simulink library "WECSim_Lib"  (R2014b)
settings: Solver=ode45  StartTime=0.0  StopTime=10.0  RelTol=1e-3
undefined symbols (not defined in the file): body, constraint, pto, simu, waves, X, Y, Z
libraries: nesl_utility x107, sm_lib x53
(part 2 of 4)

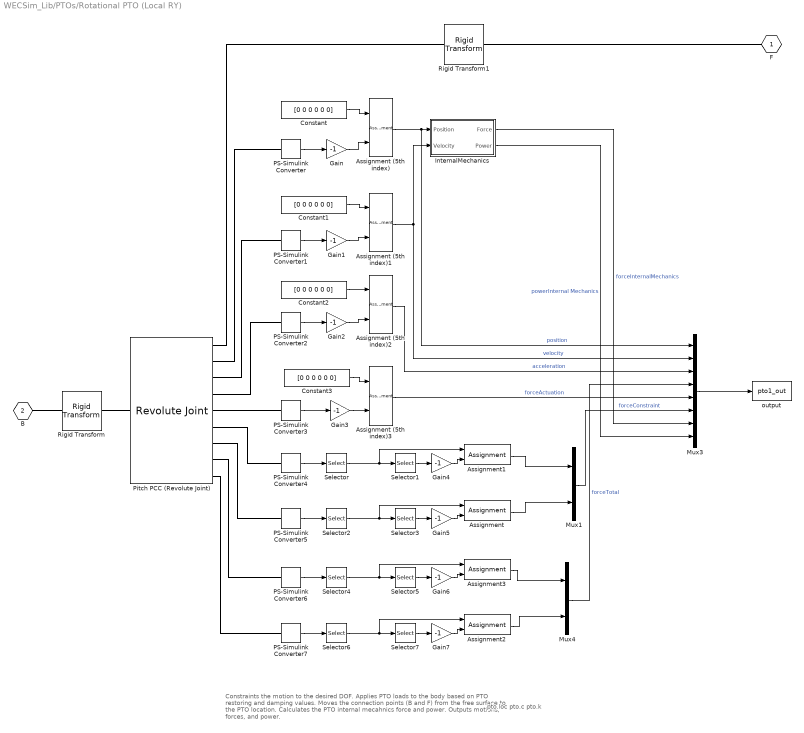
== system WECSim_Lib/PTOs/Rotational PTO (Local RY) ==
  note: Constraints the motion to the desired DOF.
      | Applies PTO loads to the body based on PTO restoring and damping values.
      | Moves the connection points (B and F) from the free surface to the PTO location.
      | Calculates the PTO internal mecahnics force and power.
      | Outputs motions, forces, and power.
  note: pto.loc
      | pto.c
      | pto.k
  Assignment{,1..3} (4 alike) : Assignment  DiagnosticForDimensions=Warning  Indices=2
  "Assignment (5th index) " : Assignment  Indices=5
  Assignment (5th index)1 : Assignment  Indices=5
  Assignment (5th index)2 : Assignment  Indices=5
  Assignment (5th index)3 : Assignment  Indices=5
  Constant{,1..3} (4 alike) : Constant  Value=[0 0 0 0 0 0]
  Gain{,1..7} (8 alike) : Gain  Gain=-1
  InternalMechanics : Subsystem
  Mux1 : Mux  Inputs=2
  Mux3 : Mux  Inputs=8
  Mux4 : Mux  Inputs=2
  PS-Simulink Converter{,1..7} (8 alike) : nesl_utility/PS-Simulink Converter  PhysicalDomain=network_engine_domain  SubClassName=ps_output  LeftPortType=input  RightPortType=output  PseudoPeriodic=off  Frequencies=[]  Unit=1  AffineConversion=off
  Pitch PCC (Revolute Joint) : sm_lib/Joints/Revolute Joint  SenseConstraintForce=on  SenseConstraintForceX=off  SenseConstraintForceY=off  SenseConstraintForceZ=off  SenseConstraintTorque=on  SenseConstraintTorqueX=off  SenseConstraintTorqueY=off  SenseConstraintTorqueZ=off  SenseTotalForce=on  SenseTotalForceX=off  SenseTotalForceY=off  SenseTotalForceZ=off  SenseTotalTorque=on  SenseTotalTorqueX=off  SenseTotalTorqueY=off  SenseTotalTorqueZ=off  CompositeWrenchDir=BaseOnFollower  CompositeWrenchFrame=BaseFrame  EquilibriumPosition=0  EquilibriumPositionUnits=deg  SpringStiffness=pto.k  SpringStiffnessUnits=N*m/rad  DampingCoefficient=pto.c  DampingCoefficientUnits=N*m/(rad/s)  TorqueActuationMode=NoTorque  MotionActuationMode=ComputedMotion  SensePosition=on  SenseVelocity=on  SenseAcceleration=on  SenseTorqueForce=on  PositionTargetValue=0  PositionTargetValueUnits=deg  PositionTargetSpecify=off  PositionTargetPriority=High  VelocityTargetValue=0  VelocityTargetValueUnits=deg/s  VelocityTargetSpecify=off  VelocityTargetPriority=High  BlockFunction=simmechanics.library.joints.revolute_joint
  Rigid Transform : sm_lib/Frames and Transforms/Rigid Transform  TranslationMethod=Cartesian  TranslationLengthUnit=m  TranslationStandardAxis=+Z  TranslationStandardOffset=0  TranslationCartesianOffset=pto.loc  TranslationROffset=0  TranslationROffsetUnits=m  TranslationZOffset=0  TranslationZOffsetUnits=m  TranslationThetaOffset=0  TranslationThetaOffsetUnits=deg  RotationMethod=StandardAxis  RotationAngleUnits=deg  RotationStandardAxis=+X  RotationAngle=90  RotationArbitraryAxis=[0 0 1]  FollAlignAxisA=+X  BaseAlignAxisA=+Y  FollAlignAxisB=+Y  BaseAlignAxisB=+Z  RotationMatrix=[1 0 0; 0 1 0; 0 0 1]  BlockFunction=simmechanics.library.frames_transforms.rigid_transform
  Rigid Transform1 : sm_lib/Frames and Transforms/Rigid Transform  TranslationMethod=Cartesian  TranslationLengthUnit=m  TranslationStandardAxis=+Z  TranslationStandardOffset=0  TranslationCartesianOffset=pto.loc  TranslationROffset=0  TranslationROffsetUnits=m  TranslationZOffset=0  TranslationZOffsetUnits=m  TranslationThetaOffset=0  TranslationThetaOffsetUnits=deg  RotationMethod=StandardAxis  RotationAngleUnits=deg  RotationStandardAxis=+X  RotationAngle=90  RotationArbitraryAxis=[0 0 1]  FollAlignAxisA=+X  BaseAlignAxisA=+Y  FollAlignAxisB=+Y  BaseAlignAxisB=+Z  RotationMatrix=[1 0 0; 0 1 0; 0 0 1]  BlockFunction=simmechanics.library.frames_transforms.rigid_transform
  Selector{,2,4,6} (4 alike) : Selector  InputPortWidth=3  Indices=[1 3 2]
  Selector{1,3,5,7} (4 alike) : Selector  InputPortWidth=3  Indices=[2]
  output : ToWorkspace  VariableName=pto1_out  SaveFormat=Structure With Time  SampleTime=-1
  F : PMIOPort  Port=1  Side=Right
  B : PMIOPort  Port=2  Side=Left
  wires:
  InternalMechanics/2(Power) -> Mux3/8  "powerInternal Mechanics"
  InternalMechanics/1(Force) -> Mux3/7  "forceInternalMechanics"
  Assignment (5th index)3/1 -> Mux3/5  "forceActuation"
  Assignment (5th index)2/1 -> Mux3/3  "acceleration"
  PS-Simulink Converter3/1 -> Gain3/1
  Gain3/1 -> Assignment (5th index)3/2
  Constant3/1 -> Assignment (5th index)3/1
  Gain2/1 -> Assignment (5th index)2/2
  Constant2/1 -> Assignment (5th index)2/1
  PS-Simulink Converter2/1 -> Gain2/1
  Assignment (5th index)1/1 -> InternalMechanics/2(Velocity), Mux3/2  "velocity"
  PS-Simulink Converter1/1 -> Gain1/1
  Gain1/1 -> Assignment (5th index)1/2
  Constant1/1 -> Assignment (5th index)1/1
  "Assignment (5th index) "/1 -> InternalMechanics/1(Position), Mux3/1  "position"
  Gain/1 -> "Assignment (5th index) "/2
  PS-Simulink Converter/1 -> Gain/1
  Constant/1 -> "Assignment (5th index) "/1
  Assignment3/1 -> Mux4/1
  Assignment2/1 -> Mux4/2
  PS-Simulink Converter7/1 -> Selector6/1
  PS-Simulink Converter6/1 -> Selector4/1
  Gain6/1 -> Assignment3/2
  Selector5/1 -> Gain6/1
  Selector4/1 -> Assignment3/1, Selector5/1
  Gain7/1 -> Assignment2/2
  Selector7/1 -> Gain7/1
  Selector6/1 -> Assignment2/1, Selector7/1
  Mux4/1 -> Mux3/4  "forceTotal"
  Mux3/1 -> output/1
  PS-Simulink Converter4/1 -> Selector/1
  PS-Simulink Converter5/1 -> Selector2/1
  Mux1/1 -> Mux3/6  "forceConstraint"
  Assignment1/1 -> Mux1/1
  Assignment/1 -> Mux1/2
  Gain4/1 -> Assignment1/2
  Selector1/1 -> Gain4/1
  Selector/1 -> Selector1/1, Assignment1/1
  Gain5/1 -> Assignment/2
  Selector3/1 -> Gain5/1
  Selector2/1 -> Selector3/1, Assignment/1
  connections:
  PS-Simulink Converter3/LConn1 -- Pitch PCC (Revolute Joint)/RConn5
  PS-Simulink Converter2/LConn1 -- Pitch PCC (Revolute Joint)/RConn4
  Pitch PCC (Revolute Joint)/RConn3 -- PS-Simulink Converter1/LConn1
  Pitch PCC (Revolute Joint)/RConn2 -- PS-Simulink Converter/LConn1
  PS-Simulink Converter4/LConn1 -- Pitch PCC (Revolute Joint)/RConn6
  PS-Simulink Converter5/LConn1 -- Pitch PCC (Revolute Joint)/RConn7
  PS-Simulink Converter6/LConn1 -- Pitch PCC (Revolute Joint)/RConn8
  PS-Simulink Converter7/LConn1 -- Pitch PCC (Revolute Joint)/RConn9
  Pitch PCC (Revolute Joint)/RConn1 -- Rigid Transform1/RConn1
  Pitch PCC (Revolute Joint)/LConn1 -- Rigid Transform/RConn1
  B/RConn1 -- Rigid Transform/LConn1
  F/RConn1 -- Rigid Transform1/LConn1

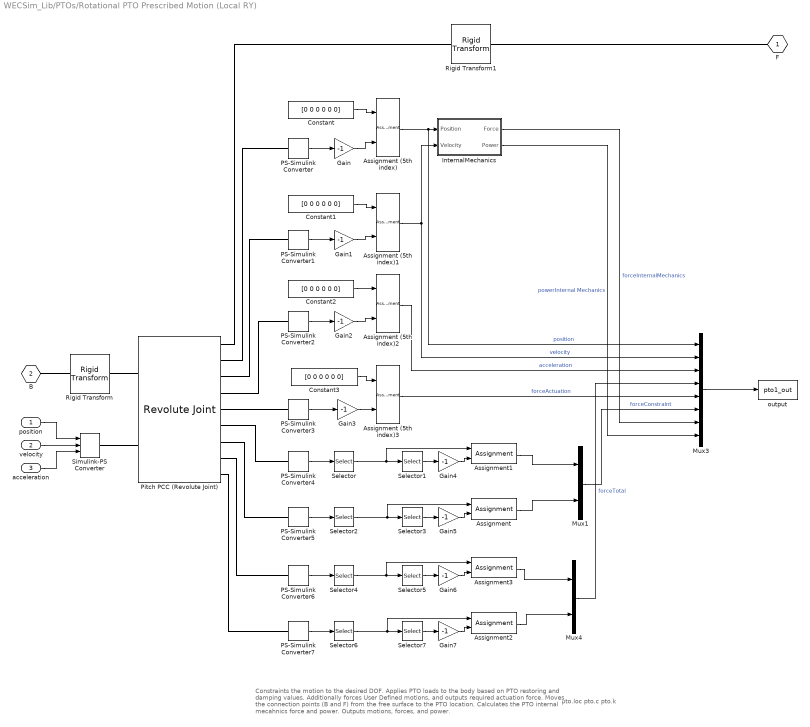
== system WECSim_Lib/PTOs/Rotational PTO Prescribed Motion (Local RY) ==
  note: pto.loc
      | pto.c
      | pto.k
  note: Constraints the motion to the desired DOF.
      | Applies PTO loads to the body based on PTO restoring and damping values.
      | Additionally forces User Defined motions, and outputs required actuation force.
      | Moves the connection points (B and F) from the free surface to the PTO location.
      | Calculates the PTO internal mecahnics force and power.
      | Outputs motions, forces, and power.
  position : Inport
  velocity : Inport  Port=2
  acceleration : Inport  Port=3
  Assignment{,1..3} (4 alike) : Assignment  DiagnosticForDimensions=Warning  Indices=2
  "Assignment (5th index) " : Assignment  Indices=5
  Assignment (5th index)1 : Assignment  Indices=5
  Assignment (5th index)2 : Assignment  Indices=5
  Assignment (5th index)3 : Assignment  Indices=5
  Constant{,1..3} (4 alike) : Constant  Value=[0 0 0 0 0 0]
  Gain{,1..7} (8 alike) : Gain  Gain=-1
  InternalMechanics : Subsystem
  Mux1 : Mux  Inputs=2
  Mux3 : Mux  Inputs=8
  Mux4 : Mux  Inputs=2
  PS-Simulink Converter{,1..7} (8 alike) : nesl_utility/PS-Simulink Converter  PhysicalDomain=network_engine_domain  SubClassName=ps_output  LeftPortType=input  RightPortType=output  PseudoPeriodic=off  Frequencies=[]  Unit=1  AffineConversion=off
  Pitch PCC (Revolute Joint) : sm_lib/Joints/Revolute Joint  SenseConstraintForce=on  SenseConstraintForceX=off  SenseConstraintForceY=off  SenseConstraintForceZ=off  SenseConstraintTorque=on  SenseConstraintTorqueX=off  SenseConstraintTorqueY=off  SenseConstraintTorqueZ=off  SenseTotalForce=on  SenseTotalForceX=off  SenseTotalForceY=off  SenseTotalForceZ=off  SenseTotalTorque=on  SenseTotalTorqueX=off  SenseTotalTorqueY=off  SenseTotalTorqueZ=off  CompositeWrenchDir=BaseOnFollower  CompositeWrenchFrame=BaseFrame  EquilibriumPosition=0  EquilibriumPositionUnits=deg  SpringStiffness=pto.k  SpringStiffnessUnits=N*m/rad  DampingCoefficient=pto.c  DampingCoefficientUnits=N*m/(rad/s)  TorqueActuationMode=ComputedTorque  MotionActuationMode=InputMotion  SensePosition=on  SenseVelocity=on  SenseAcceleration=on  SenseTorqueForce=on  PositionTargetValue=0  PositionTargetValueUnits=deg  PositionTargetSpecify=off  PositionTargetPriority=High  VelocityTargetValue=0  VelocityTargetValueUnits=deg/s  VelocityTargetSpecify=off  VelocityTargetPriority=High  BlockFunction=simmechanics.library.joints.revolute_joint
  Rigid Transform : sm_lib/Frames and Transforms/Rigid Transform  TranslationMethod=Cartesian  TranslationLengthUnit=m  TranslationStandardAxis=+Z  TranslationStandardOffset=0  TranslationCartesianOffset=pto.loc  TranslationROffset=0  TranslationROffsetUnits=m  TranslationZOffset=0  TranslationZOffsetUnits=m  TranslationThetaOffset=0  TranslationThetaOffsetUnits=deg  RotationMethod=StandardAxis  RotationAngleUnits=deg  RotationStandardAxis=+X  RotationAngle=90  RotationArbitraryAxis=[0 0 1]  FollAlignAxisA=+X  BaseAlignAxisA=+Y  FollAlignAxisB=+Y  BaseAlignAxisB=+Z  RotationMatrix=[1 0 0; 0 1 0; 0 0 1]  BlockFunction=simmechanics.library.frames_transforms.rigid_transform
  Rigid Transform1 : sm_lib/Frames and Transforms/Rigid Transform  TranslationMethod=Cartesian  TranslationLengthUnit=m  TranslationStandardAxis=+Z  TranslationStandardOffset=0  TranslationCartesianOffset=pto.loc  TranslationROffset=0  TranslationROffsetUnits=m  TranslationZOffset=0  TranslationZOffsetUnits=m  TranslationThetaOffset=0  TranslationThetaOffsetUnits=deg  RotationMethod=StandardAxis  RotationAngleUnits=deg  RotationStandardAxis=+X  RotationAngle=90  RotationArbitraryAxis=[0 0 1]  FollAlignAxisA=+X  BaseAlignAxisA=+Y  FollAlignAxisB=+Y  BaseAlignAxisB=+Z  RotationMatrix=[1 0 0; 0 1 0; 0 0 1]  BlockFunction=simmechanics.library.frames_transforms.rigid_transform
  Selector{,2,4,6} (4 alike) : Selector  InputPortWidth=3  Indices=[1 3 2]
  Selector{1,3,5,7} (4 alike) : Selector  InputPortWidth=3  Indices=[2]
  Simulink-PS Converter : nesl_utility/Simulink-PS Converter  PhysicalDomain=network_engine_domain  SubClassName=ps_input  LeftPortType=input  RightPortType=output  PseudoPeriodic=off  Frequencies=[]  NoiseDistribution=none  NoiseParameters=[]  Unit=1  AffineConversion=off  InputFiltering=derivs  SimscapeFilterOrder=2  InputFilterTimeConstant=0.001  UdotUserProvided=2
  output : ToWorkspace  VariableName=pto1_out  SaveFormat=Structure With Time  SampleTime=-1
  F : PMIOPort  Port=1  Side=Left
  B : PMIOPort  Port=2  Side=Right
  wires:
  position/1 -> Simulink-PS Converter/1
  velocity/1 -> Simulink-PS Converter/2
  acceleration/1 -> Simulink-PS Converter/3
  Selector2/1 -> Assignment/1, Selector3/1
  Selector3/1 -> Gain5/1
  Gain5/1 -> Assignment/2
  Selector/1 -> Assignment1/1, Selector1/1
  Selector1/1 -> Gain4/1
  Gain4/1 -> Assignment1/2
  Assignment/1 -> Mux1/2
  Assignment1/1 -> Mux1/1
  Mux1/1 -> Mux3/6  "forceConstraint"
  PS-Simulink Converter5/1 -> Selector2/1
  PS-Simulink Converter4/1 -> Selector/1
  Mux3/1 -> output/1
  Mux4/1 -> Mux3/4  "forceTotal"
  Selector6/1 -> Selector7/1, Assignment2/1
  Selector7/1 -> Gain7/1
  Gain7/1 -> Assignment2/2
  Selector4/1 -> Selector5/1, Assignment3/1
  Selector5/1 -> Gain6/1
  Gain6/1 -> Assignment3/2
  PS-Simulink Converter6/1 -> Selector4/1
  PS-Simulink Converter7/1 -> Selector6/1
  Assignment2/1 -> Mux4/2
  Assignment3/1 -> Mux4/1
  Constant/1 -> "Assignment (5th index) "/1
  PS-Simulink Converter/1 -> Gain/1
  Gain/1 -> "Assignment (5th index) "/2
  "Assignment (5th index) "/1 -> Mux3/1, InternalMechanics/1(Position)  "position"
  Constant1/1 -> Assignment (5th index)1/1
  Gain1/1 -> Assignment (5th index)1/2
  PS-Simulink Converter1/1 -> Gain1/1
  Assignment (5th index)1/1 -> Mux3/2, InternalMechanics/2(Velocity)  "velocity"
  PS-Simulink Converter2/1 -> Gain2/1
  Constant2/1 -> Assignment (5th index)2/1
  Gain2/1 -> Assignment (5th index)2/2
  Constant3/1 -> Assignment (5th index)3/1
  Gain3/1 -> Assignment (5th index)3/2
  PS-Simulink Converter3/1 -> Gain3/1
  Assignment (5th index)2/1 -> Mux3/3  "acceleration"
  Assignment (5th index)3/1 -> Mux3/5  "forceActuation"
  InternalMechanics/1(Force) -> Mux3/7  "forceInternalMechanics"
  InternalMechanics/2(Power) -> Mux3/8  "powerInternal Mechanics"
  connections:
  Pitch PCC (Revolute Joint)/LConn2 -- Simulink-PS Converter/RConn1
  PS-Simulink Converter3/LConn1 -- Pitch PCC (Revolute Joint)/RConn5
  PS-Simulink Converter6/LConn1 -- Pitch PCC (Revolute Joint)/RConn8
  PS-Simulink Converter7/LConn1 -- Pitch PCC (Revolute Joint)/RConn9
  F/RConn1 -- Rigid Transform1/LConn1
  Pitch PCC (Revolute Joint)/RConn3 -- PS-Simulink Converter1/LConn1
  Pitch PCC (Revolute Joint)/RConn2 -- PS-Simulink Converter/LConn1
  Pitch PCC (Revolute Joint)/LConn1 -- Rigid Transform/RConn1
  B/RConn1 -- Rigid Transform/LConn1
  Pitch PCC (Revolute Joint)/RConn1 -- Rigid Transform1/RConn1
  PS-Simulink Converter2/LConn1 -- Pitch PCC (Revolute Joint)/RConn4
  PS-Simulink Converter4/LConn1 -- Pitch PCC (Revolute Joint)/RConn6
  PS-Simulink Converter5/LConn1 -- Pitch PCC (Revolute Joint)/RConn7

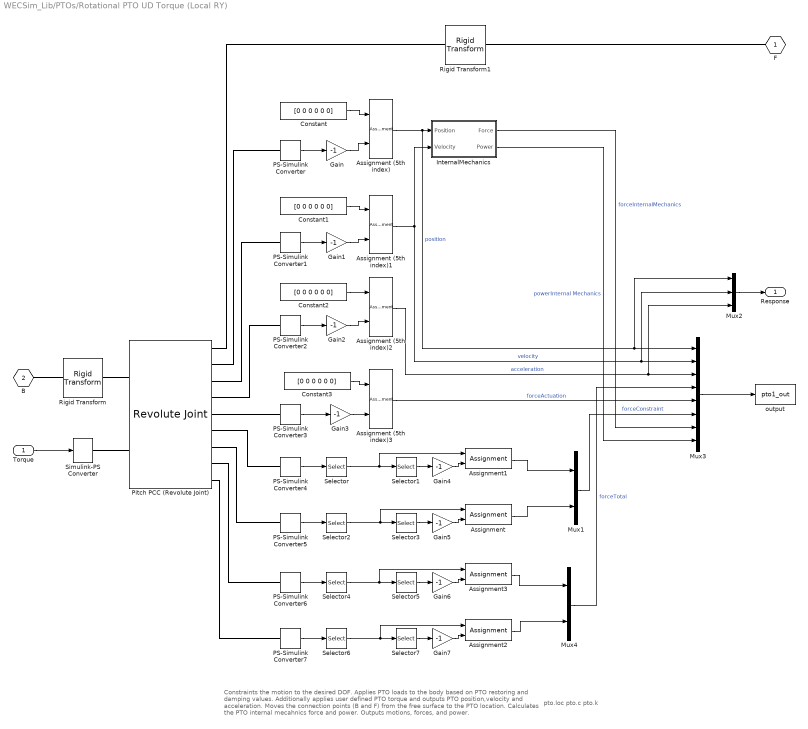
== system WECSim_Lib/PTOs/Rotational PTO UD Torque (Local RY) ==
  note: Constraints the motion to the desired DOF.
      | Applies PTO loads to the body based on PTO restoring and damping values.
      | Additionally applies user defined PTO torque and outputs PTO position,velocity and acceleration.
      | Moves the connection points (B and F) from the free surface to the PTO location.
      | Calculates the PTO internal mecahnics force and power.
      | Outputs motions, forces, and power.
  note: pto.loc
      | pto.c
      | pto.k
  Torque : Inport
  Assignment{,1..3} (4 alike) : Assignment  DiagnosticForDimensions=Warning  Indices=2
  "Assignment (5th index) " : Assignment  Indices=5
  Assignment (5th index)1 : Assignment  Indices=5
  Assignment (5th index)2 : Assignment  Indices=5
  Assignment (5th index)3 : Assignment  Indices=5
  Constant{,1..3} (4 alike) : Constant  Value=[0 0 0 0 0 0]
  Gain{,1..7} (8 alike) : Gain  Gain=-1
  InternalMechanics : Subsystem
  Mux1 : Mux  Inputs=2
  Mux2 : Mux  Inputs=3
  Mux3 : Mux  Inputs=8
  Mux4 : Mux  Inputs=2
  PS-Simulink Converter{,1..7} (8 alike) : nesl_utility/PS-Simulink Converter  PhysicalDomain=network_engine_domain  SubClassName=ps_output  LeftPortType=input  RightPortType=output  PseudoPeriodic=off  Frequencies=[]  Unit=1  AffineConversion=off
  Pitch PCC (Revolute Joint) : sm_lib/Joints/Revolute Joint  SenseConstraintForce=on  SenseConstraintForceX=off  SenseConstraintForceY=off  SenseConstraintForceZ=off  SenseConstraintTorque=on  SenseConstraintTorqueX=off  SenseConstraintTorqueY=off  SenseConstraintTorqueZ=off  SenseTotalForce=on  SenseTotalForceX=off  SenseTotalForceY=off  SenseTotalForceZ=off  SenseTotalTorque=on  SenseTotalTorqueX=off  SenseTotalTorqueY=off  SenseTotalTorqueZ=off  CompositeWrenchDir=BaseOnFollower  CompositeWrenchFrame=BaseFrame  EquilibriumPosition=0  EquilibriumPositionUnits=deg  SpringStiffness=pto.k  SpringStiffnessUnits=N*m/rad  DampingCoefficient=pto.c  DampingCoefficientUnits=N*m/(rad/s)  TorqueActuationMode=InputTorque  MotionActuationMode=ComputedMotion  SensePosition=on  SenseVelocity=on  SenseAcceleration=on  SenseTorqueForce=on  PositionTargetValue=0  PositionTargetValueUnits=deg  PositionTargetSpecify=off  PositionTargetPriority=High  VelocityTargetValue=0  VelocityTargetValueUnits=deg/s  VelocityTargetSpecify=off  VelocityTargetPriority=High  BlockFunction=simmechanics.library.joints.revolute_joint
  Rigid Transform : sm_lib/Frames and Transforms/Rigid Transform  TranslationMethod=Cartesian  TranslationLengthUnit=m  TranslationStandardAxis=+Z  TranslationStandardOffset=0  TranslationCartesianOffset=pto.loc  TranslationROffset=0  TranslationROffsetUnits=m  TranslationZOffset=0  TranslationZOffsetUnits=m  TranslationThetaOffset=0  TranslationThetaOffsetUnits=deg  RotationMethod=StandardAxis  RotationAngleUnits=deg  RotationStandardAxis=+X  RotationAngle=90  RotationArbitraryAxis=[0 0 1]  FollAlignAxisA=+X  BaseAlignAxisA=+Y  FollAlignAxisB=+Y  BaseAlignAxisB=+Z  RotationMatrix=[1 0 0; 0 1 0; 0 0 1]  BlockFunction=simmechanics.library.frames_transforms.rigid_transform
  Rigid Transform1 : sm_lib/Frames and Transforms/Rigid Transform  TranslationMethod=Cartesian  TranslationLengthUnit=m  TranslationStandardAxis=+Z  TranslationStandardOffset=0  TranslationCartesianOffset=pto.loc  TranslationROffset=0  TranslationROffsetUnits=m  TranslationZOffset=0  TranslationZOffsetUnits=m  TranslationThetaOffset=0  TranslationThetaOffsetUnits=deg  RotationMethod=StandardAxis  RotationAngleUnits=deg  RotationStandardAxis=+X  RotationAngle=90  RotationArbitraryAxis=[0 0 1]  FollAlignAxisA=+X  BaseAlignAxisA=+Y  FollAlignAxisB=+Y  BaseAlignAxisB=+Z  RotationMatrix=[1 0 0; 0 1 0; 0 0 1]  BlockFunction=simmechanics.library.frames_transforms.rigid_transform
  Selector{,2,4,6} (4 alike) : Selector  InputPortWidth=3  Indices=[1 3 2]
  Selector{1,3,5,7} (4 alike) : Selector  InputPortWidth=3  Indices=[2]
  Simulink-PS Converter : nesl_utility/Simulink-PS Converter  PhysicalDomain=network_engine_domain  SubClassName=ps_input  LeftPortType=input  RightPortType=output  PseudoPeriodic=off  Frequencies=[]  NoiseDistribution=none  NoiseParameters=[]  Unit=1  AffineConversion=off  InputFiltering=off  SimscapeFilterOrder=1  InputFilterTimeConstant=0.001  UdotUserProvided=1
  output : ToWorkspace  VariableName=pto1_out  SaveFormat=Structure With Time  SampleTime=-1
  F : PMIOPort  Port=1  Side=Left
  B : PMIOPort  Port=2  Side=Right
  Response : Outport
  wires:
  Mux2/1 -> Response/1
  Torque/1 -> Simulink-PS Converter/1
  Selector2/1 -> Assignment/1, Selector3/1
  Selector3/1 -> Gain5/1
  Gain5/1 -> Assignment/2
  Selector/1 -> Assignment1/1, Selector1/1
  Selector1/1 -> Gain4/1
  Gain4/1 -> Assignment1/2
  Assignment/1 -> Mux1/2
  Assignment1/1 -> Mux1/1
  Mux1/1 -> Mux3/6  "forceConstraint"
  PS-Simulink Converter5/1 -> Selector2/1
  PS-Simulink Converter4/1 -> Selector/1
  Mux3/1 -> output/1
  Mux4/1 -> Mux3/4  "forceTotal"
  Selector6/1 -> Selector7/1, Assignment2/1
  Selector7/1 -> Gain7/1
  Gain7/1 -> Assignment2/2
  Selector4/1 -> Selector5/1, Assignment3/1
  Selector5/1 -> Gain6/1
  Gain6/1 -> Assignment3/2
  PS-Simulink Converter6/1 -> Selector4/1
  PS-Simulink Converter7/1 -> Selector6/1
  Assignment2/1 -> Mux4/2
  Assignment3/1 -> Mux4/1
  Constant/1 -> "Assignment (5th index) "/1
  PS-Simulink Converter/1 -> Gain/1
  Gain/1 -> "Assignment (5th index) "/2
  "Assignment (5th index) "/1 -> Mux3/1, Mux2/1, InternalMechanics/1(Position)  "position"
  Constant1/1 -> Assignment (5th index)1/1
  Gain1/1 -> Assignment (5th index)1/2
  PS-Simulink Converter1/1 -> Gain1/1
  Assignment (5th index)1/1 -> Mux3/2, Mux2/2, InternalMechanics/2(Velocity)  "velocity"
  PS-Simulink Converter2/1 -> Gain2/1
  Constant2/1 -> Assignment (5th index)2/1
  Gain2/1 -> Assignment (5th index)2/2
  Constant3/1 -> Assignment (5th index)3/1
  Gain3/1 -> Assignment (5th index)3/2
  PS-Simulink Converter3/1 -> Gain3/1
  Assignment (5th index)2/1 -> Mux2/3, Mux3/3  "acceleration"
  Assignment (5th index)3/1 -> Mux3/5  "forceActuation"
  InternalMechanics/1(Force) -> Mux3/7  "forceInternalMechanics"
  InternalMechanics/2(Power) -> Mux3/8  "powerInternal Mechanics"
  connections:
  Simulink-PS Converter/RConn1 -- Pitch PCC (Revolute Joint)/LConn2
  PS-Simulink Converter3/LConn1 -- Pitch PCC (Revolute Joint)/RConn5
  PS-Simulink Converter6/LConn1 -- Pitch PCC (Revolute Joint)/RConn8
  PS-Simulink Converter7/LConn1 -- Pitch PCC (Revolute Joint)/RConn9
  F/RConn1 -- Rigid Transform1/LConn1
  Pitch PCC (Revolute Joint)/RConn3 -- PS-Simulink Converter1/LConn1
  Pitch PCC (Revolute Joint)/RConn2 -- PS-Simulink Converter/LConn1
  Pitch PCC (Revolute Joint)/LConn1 -- Rigid Transform/RConn1
  B/RConn1 -- Rigid Transform/LConn1
  Pitch PCC (Revolute Joint)/RConn1 -- Rigid Transform1/RConn1
  PS-Simulink Converter2/LConn1 -- Pitch PCC (Revolute Joint)/RConn4
  PS-Simulink Converter4/LConn1 -- Pitch PCC (Revolute Joint)/RConn6
  PS-Simulink Converter5/LConn1 -- Pitch PCC (Revolute Joint)/RConn7

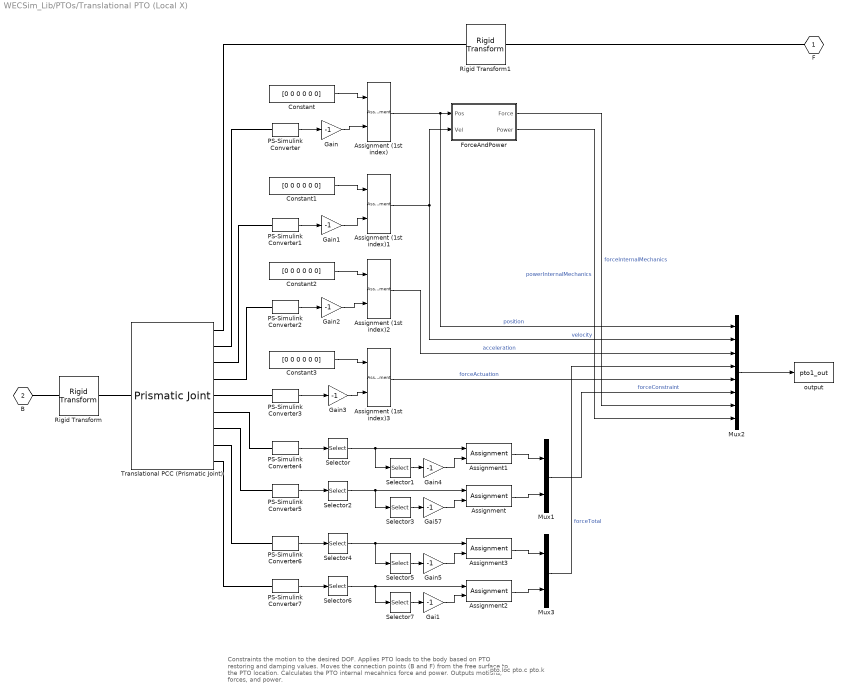
== system WECSim_Lib/PTOs/Translational PTO (Local X) ==
  note: Constraints the motion to the desired DOF.
      | Applies PTO loads to the body based on PTO restoring and damping values.
      | Moves the connection points (B and F) from the free surface to the PTO location.
      | Calculates the PTO internal mecahnics force and power.
      | Outputs motions, forces, and power.
  note: pto.loc
      | pto.c
      | pto.k
  Assignment{,1..3} (4 alike) : Assignment  DiagnosticForDimensions=Warning
  "Assignment (1st index) " : Assignment
  Assignment (1st index)1 : Assignment
  Assignment (1st index)2 : Assignment
  Assignment (1st index)3 : Assignment
  Constant{,1..3} (4 alike) : Constant  Value=[0 0 0 0 0 0]
  ForceAndPower : Subsystem
  Gai1 : Gain  Gain=-1
  Gai57 : Gain  Gain=-1
  Gain{,1..5} (6 alike) : Gain  Gain=-1
  Mux1 : Mux  Inputs=2
  Mux2 : Mux  Inputs=8
  Mux3 : Mux  Inputs=2
  PS-Simulink Converter{,1..7} (8 alike) : nesl_utility/PS-Simulink Converter  PhysicalDomain=network_engine_domain  SubClassName=ps_output  LeftPortType=input  RightPortType=output  PseudoPeriodic=off  Frequencies=[]  Unit=1  AffineConversion=off
  Rigid Transform : sm_lib/Frames and Transforms/Rigid Transform  TranslationMethod=Cartesian  TranslationLengthUnit=m  TranslationStandardAxis=+Z  TranslationStandardOffset=0  TranslationCartesianOffset=pto.loc  TranslationROffset=0  TranslationROffsetUnits=m  TranslationZOffset=0  TranslationZOffsetUnits=m  TranslationThetaOffset=0  TranslationThetaOffsetUnits=deg  RotationMethod=StandardAxis  RotationAngleUnits=deg  RotationStandardAxis=+Y  RotationAngle=90  RotationArbitraryAxis=[0 0 1]  FollAlignAxisA=+X  BaseAlignAxisA=+Y  FollAlignAxisB=+Y  BaseAlignAxisB=+Z  RotationMatrix=[1 0 0; 0 1 0; 0 0 1]  BlockFunction=simmechanics.library.frames_transforms.rigid_transform
  Rigid Transform1 : sm_lib/Frames and Transforms/Rigid Transform  TranslationMethod=Cartesian  TranslationLengthUnit=m  TranslationStandardAxis=+Z  TranslationStandardOffset=0  TranslationCartesianOffset=pto.loc  TranslationROffset=0  TranslationROffsetUnits=m  TranslationZOffset=0  TranslationZOffsetUnits=m  TranslationThetaOffset=0  TranslationThetaOffsetUnits=deg  RotationMethod=StandardAxis  RotationAngleUnits=deg  RotationStandardAxis=+Y  RotationAngle=90  RotationArbitraryAxis=[0 0 1]  FollAlignAxisA=+X  BaseAlignAxisA=+Y  FollAlignAxisB=+Y  BaseAlignAxisB=+Z  RotationMatrix=[1 0 0; 0 1 0; 0 0 1]  BlockFunction=simmechanics.library.frames_transforms.rigid_transform
  Selector{,2,4,6} (4 alike) : Selector  InputPortWidth=3  Indices=[3 2 1]
  Selector{1,3,5,7} (4 alike) : Selector  InputPortWidth=3  Indices=[3]
  Translational PCC (Prismatic Joint) : sm_lib/Joints/Prismatic Joint  SenseConstraintForce=on  SenseConstraintForceX=off  SenseConstraintForceY=off  SenseConstraintForceZ=off  SenseConstraintTorque=on  SenseConstraintTorqueX=off  SenseConstraintTorqueY=off  SenseConstraintTorqueZ=off  SenseTotalForce=on  SenseTotalForceX=off  SenseTotalForceY=off  SenseTotalForceZ=off  SenseTotalTorque=on  SenseTotalTorqueX=off  SenseTotalTorqueY=off  SenseTotalTorqueZ=off  CompositeWrenchDir=BaseOnFollower  CompositeWrenchFrame=BaseFrame  EquilibriumPosition=0  EquilibriumPositionUnits=m  SpringStiffness=pto.k  SpringStiffnessUnits=N/m  DampingCoefficient=pto.c  DampingCoefficientUnits=N/(m/s)  TorqueActuationMode=NoTorque  MotionActuationMode=ComputedMotion  SensePosition=on  SenseVelocity=on  SenseAcceleration=on  SenseTorqueForce=on  PositionTargetValue=0  PositionTargetValueUnits=m  PositionTargetSpecify=off  PositionTargetPriority=High  VelocityTargetValue=0  VelocityTargetValueUnits=m/s  VelocityTargetSpecify=off  VelocityTargetPriority=High  BlockFunction=simmechanics.library.joints.prismatic_joint
  output : ToWorkspace  VariableName=pto1_out  SaveFormat=Structure With Time  SampleTime=-1
  F : PMIOPort  Port=1  Side=Left
  B : PMIOPort  Port=2  Side=Right
  wires:
  Assignment2/1 -> Mux3/2
  Assignment3/1 -> Mux3/1
  PS-Simulink Converter7/1 -> Selector6/1
  PS-Simulink Converter6/1 -> Selector4/1
  Gain5/1 -> Assignment3/2
  Selector5/1 -> Gain5/1
  Selector4/1 -> Selector5/1, Assignment3/1
  Gai1/1 -> Assignment2/2
  Selector7/1 -> Gai1/1
  Selector6/1 -> Selector7/1, Assignment2/1
  Assignment/1 -> Mux1/2
  Assignment1/1 -> Mux1/1
  Gain3/1 -> Assignment (1st index)3/2
  PS-Simulink Converter3/1 -> Gain3/1
  PS-Simulink Converter2/1 -> Gain2/1
  Gain2/1 -> Assignment (1st index)2/2
  Constant3/1 -> Assignment (1st index)3/1
  Constant2/1 -> Assignment (1st index)2/1
  Gain1/1 -> Assignment (1st index)1/2
  Constant1/1 -> Assignment (1st index)1/1
  Gain/1 -> "Assignment (1st index) "/2
  PS-Simulink Converter/1 -> Gain/1
  Constant/1 -> "Assignment (1st index) "/1
  PS-Simulink Converter1/1 -> Gain1/1
  PS-Simulink Converter5/1 -> Selector2/1
  PS-Simulink Converter4/1 -> Selector/1
  Mux2/1 -> output/1
  Mux1/1 -> Mux2/6  "forceConstraint"
  Mux3/1 -> Mux2/4  "forceTotal"
  Assignment (1st index)3/1 -> Mux2/5  "forceActuation"
  "Assignment (1st index) "/1 -> ForceAndPower/1(Pos), Mux2/1  "position"
  Assignment (1st index)1/1 -> ForceAndPower/2(Vel), Mux2/2  "velocity"
  Assignment (1st index)2/1 -> Mux2/3  "acceleration"
  ForceAndPower/1(Force) -> Mux2/7  "forceInternalMechanics"
  ForceAndPower/2(Power) -> Mux2/8  "powerInternalMechanics"
  Gain4/1 -> Assignment1/2
  Selector1/1 -> Gain4/1
  Selector/1 -> Assignment1/1, Selector1/1
  Gai57/1 -> Assignment/2
  Selector3/1 -> Gai57/1
  Selector2/1 -> Assignment/1, Selector3/1
  connections:
  PS-Simulink Converter7/LConn1 -- Translational PCC (Prismatic Joint)/RConn9
  Translational PCC (Prismatic Joint)/RConn8 -- PS-Simulink Converter6/LConn1
  Translational PCC (Prismatic Joint)/RConn5 -- PS-Simulink Converter3/LConn1
  Translational PCC (Prismatic Joint)/RConn1 -- Rigid Transform1/RConn1
  Translational PCC (Prismatic Joint)/RConn4 -- PS-Simulink Converter2/LConn1
  Translational PCC (Prismatic Joint)/RConn3 -- PS-Simulink Converter1/LConn1
  Translational PCC (Prismatic Joint)/RConn2 -- PS-Simulink Converter/LConn1
  PS-Simulink Converter5/LConn1 -- Translational PCC (Prismatic Joint)/RConn7
  PS-Simulink Converter4/LConn1 -- Translational PCC (Prismatic Joint)/RConn6
  Rigid Transform1/LConn1 -- F/RConn1
  Rigid Transform/RConn1 -- Translational PCC (Prismatic Joint)/LConn1
  Rigid Transform/LConn1 -- B/RConn1

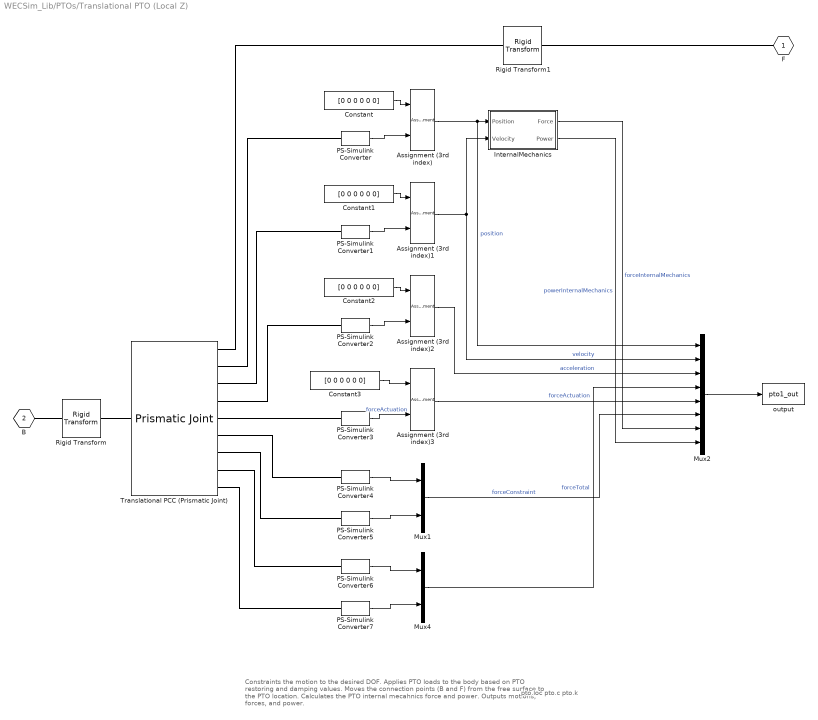
== system WECSim_Lib/PTOs/Translational PTO (Local Z) ==
  note: Constraints the motion to the desired DOF.
      | Applies PTO loads to the body based on PTO restoring and damping values.
      | Moves the connection points (B and F) from the free surface to the PTO location.
      | Calculates the PTO internal mecahnics force and power.
      | Outputs motions, forces, and power.
  note: pto.loc
      | pto.c
      | pto.k
  "Assignment (3rd index) " : Assignment  Indices=3
  Assignment (3rd index)1 : Assignment  Indices=3
  Assignment (3rd index)2 : Assignment  Indices=3
  Assignment (3rd index)3 : Assignment  Indices=3
  Constant{,1..3} (4 alike) : Constant  Value=[0 0 0 0 0 0]
  InternalMechanics : Subsystem
  Mux1 : Mux  Inputs=2
  Mux2 : Mux  Inputs=8
  Mux4 : Mux  Inputs=2
  PS-Simulink Converter{,1..7} (8 alike) : nesl_utility/PS-Simulink Converter  PhysicalDomain=network_engine_domain  SubClassName=ps_output  LeftPortType=input  RightPortType=output  PseudoPeriodic=off  Frequencies=[]  Unit=1  AffineConversion=off
  Rigid Transform : sm_lib/Frames and Transforms/Rigid Transform  TranslationMethod=Cartesian  TranslationLengthUnit=m  TranslationStandardAxis=+Z  TranslationStandardOffset=0  TranslationCartesianOffset=pto.loc  TranslationROffset=0  TranslationROffsetUnits=m  TranslationZOffset=0  TranslationZOffsetUnits=m  TranslationThetaOffset=0  TranslationThetaOffsetUnits=deg  RotationMethod=None  RotationAngleUnits=deg  RotationStandardAxis=+X  RotationAngle=90  RotationArbitraryAxis=[0 0 1]  FollAlignAxisA=+X  BaseAlignAxisA=+Y  FollAlignAxisB=+Y  BaseAlignAxisB=+Z  RotationMatrix=[1 0 0; 0 1 0; 0 0 1]  BlockFunction=simmechanics.library.frames_transforms.rigid_transform
  Rigid Transform1 : sm_lib/Frames and Transforms/Rigid Transform  TranslationMethod=Cartesian  TranslationLengthUnit=m  TranslationStandardAxis=+Z  TranslationStandardOffset=0  TranslationCartesianOffset=pto.loc  TranslationROffset=0  TranslationROffsetUnits=m  TranslationZOffset=0  TranslationZOffsetUnits=m  TranslationThetaOffset=0  TranslationThetaOffsetUnits=deg  RotationMethod=None  RotationAngleUnits=deg  RotationStandardAxis=+X  RotationAngle=90  RotationArbitraryAxis=[0 0 1]  FollAlignAxisA=+X  BaseAlignAxisA=+Y  FollAlignAxisB=+Y  BaseAlignAxisB=+Z  RotationMatrix=[1 0 0; 0 1 0; 0 0 1]  BlockFunction=simmechanics.library.frames_transforms.rigid_transform
  Translational PCC (Prismatic Joint) : sm_lib/Joints/Prismatic Joint  SenseConstraintForce=on  SenseConstraintForceX=off  SenseConstraintForceY=off  SenseConstraintForceZ=off  SenseConstraintTorque=on  SenseConstraintTorqueX=off  SenseConstraintTorqueY=off  SenseConstraintTorqueZ=off  SenseTotalForce=on  SenseTotalForceX=off  SenseTotalForceY=off  SenseTotalForceZ=off  SenseTotalTorque=on  SenseTotalTorqueX=off  SenseTotalTorqueY=off  SenseTotalTorqueZ=off  CompositeWrenchDir=BaseOnFollower  CompositeWrenchFrame=BaseFrame  EquilibriumPosition=0  EquilibriumPositionUnits=m  SpringStiffness=pto.k  SpringStiffnessUnits=N/m  DampingCoefficient=pto.c  DampingCoefficientUnits=N/(m/s)  TorqueActuationMode=NoTorque  MotionActuationMode=ComputedMotion  SensePosition=on  SenseVelocity=on  SenseAcceleration=on  SenseTorqueForce=on  PositionTargetValue=0  PositionTargetValueUnits=m  PositionTargetSpecify=off  PositionTargetPriority=High  VelocityTargetValue=0  VelocityTargetValueUnits=m/s  VelocityTargetSpecify=off  VelocityTargetPriority=High  BlockFunction=simmechanics.library.joints.prismatic_joint
  output : ToWorkspace  VariableName=pto1_out  SaveFormat=Structure With Time  SampleTime=-1
  F : PMIOPort  Port=1  Side=Left
  B : PMIOPort  Port=2  Side=Right
  wires:
  PS-Simulink Converter3/1 -> Assignment (3rd index)3/2  "forceActuation"
  Constant3/1 -> Assignment (3rd index)3/1
  InternalMechanics/2(Power) -> Mux2/8  "powerInternalMechanics"
  InternalMechanics/1(Force) -> Mux2/7  "forceInternalMechanics"
  PS-Simulink Converter2/1 -> Assignment (3rd index)2/2
  Constant2/1 -> Assignment (3rd index)2/1
  PS-Simulink Converter1/1 -> Assignment (3rd index)1/2
  Constant1/1 -> Assignment (3rd index)1/1
  PS-Simulink Converter/1 -> "Assignment (3rd index) "/2
  Constant/1 -> "Assignment (3rd index) "/1
  Assignment (3rd index)2/1 -> Mux2/3  "acceleration"
  Assignment (3rd index)1/1 -> InternalMechanics/2(Velocity), Mux2/2  "velocity"
  "Assignment (3rd index) "/1 -> InternalMechanics/1(Position), Mux2/1  "position"
  Assignment (3rd index)3/1 -> Mux2/5  "forceActuation"
  PS-Simulink Converter7/1 -> Mux4/2
  PS-Simulink Converter6/1 -> Mux4/1
  PS-Simulink Converter5/1 -> Mux1/2
  PS-Simulink Converter4/1 -> Mux1/1
  Mux4/1 -> Mux2/4  "forceTotal"
  Mux1/1 -> Mux2/6  "forceConstraint"
  Mux2/1 -> output/1
  connections:
  Translational PCC (Prismatic Joint)/RConn6 -- PS-Simulink Converter4/LConn1
  Translational PCC (Prismatic Joint)/RConn2 -- PS-Simulink Converter/LConn1
  Translational PCC (Prismatic Joint)/RConn8 -- PS-Simulink Converter6/LConn1
  Rigid Transform1/LConn1 -- F/RConn1
  Translational PCC (Prismatic Joint)/RConn3 -- PS-Simulink Converter1/LConn1
  Translational PCC (Prismatic Joint)/RConn7 -- PS-Simulink Converter5/LConn1
  Translational PCC (Prismatic Joint)/RConn4 -- PS-Simulink Converter2/LConn1
  Translational PCC (Prismatic Joint)/RConn1 -- Rigid Transform1/RConn1
  Translational PCC (Prismatic Joint)/RConn9 -- PS-Simulink Converter7/LConn1
  Translational PCC (Prismatic Joint)/RConn5 -- PS-Simulink Converter3/LConn1
  B/RConn1 -- Rigid Transform/LConn1
  Rigid Transform/RConn1 -- Translational PCC (Prismatic Joint)/LConn1

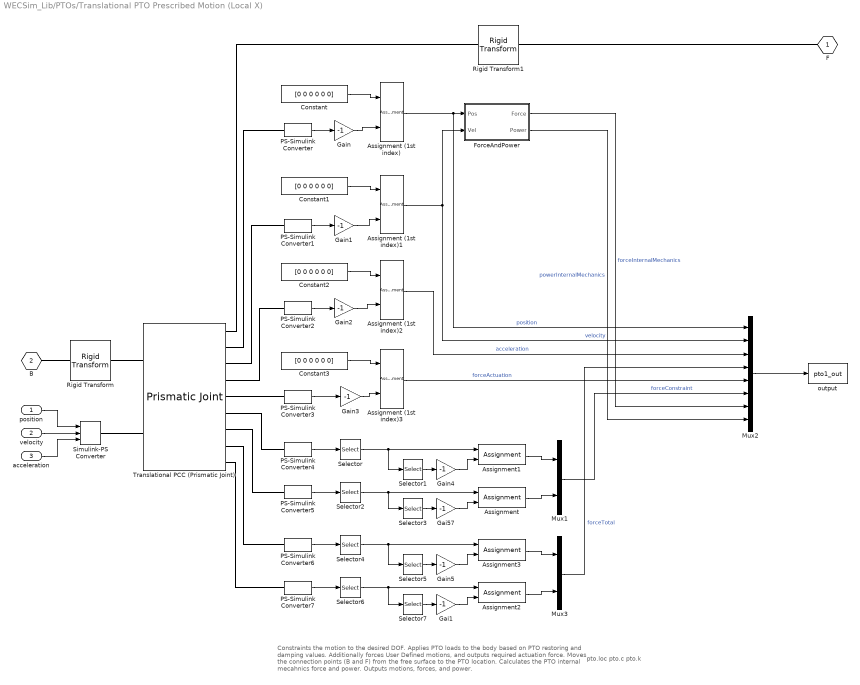
== system WECSim_Lib/PTOs/Translational PTO Prescribed Motion (Local X) ==
  note: pto.loc
      | pto.c
      | pto.k
  note: Constraints the motion to the desired DOF.
      | Applies PTO loads to the body based on PTO restoring and damping values.
      | Additionally forces User Defined motions, and outputs required actuation force.
      | Moves the connection points (B and F) from the free surface to the PTO location.
      | Calculates the PTO internal mecahnics force and power.
      | Outputs motions, forces, and power.
  position : Inport
  velocity : Inport  Port=2
  acceleration : Inport  Port=3
  Assignment{,1..3} (4 alike) : Assignment  DiagnosticForDimensions=Warning
  "Assignment (1st index) " : Assignment
  Assignment (1st index)1 : Assignment
  Assignment (1st index)2 : Assignment
  Assignment (1st index)3 : Assignment
  Constant{,1..3} (4 alike) : Constant  Value=[0 0 0 0 0 0]
  ForceAndPower : Subsystem
  Gai1 : Gain  Gain=-1
  Gai57 : Gain  Gain=-1
  Gain{,1..5} (6 alike) : Gain  Gain=-1
  Mux1 : Mux  Inputs=2
  Mux2 : Mux  Inputs=8
  Mux3 : Mux  Inputs=2
  PS-Simulink Converter{,1..7} (8 alike) : nesl_utility/PS-Simulink Converter  PhysicalDomain=network_engine_domain  SubClassName=ps_output  LeftPortType=input  RightPortType=output  PseudoPeriodic=off  Frequencies=[]  Unit=1  AffineConversion=off
  Rigid Transform : sm_lib/Frames and Transforms/Rigid Transform  TranslationMethod=Cartesian  TranslationLengthUnit=m  TranslationStandardAxis=+Z  TranslationStandardOffset=0  TranslationCartesianOffset=pto.loc  TranslationROffset=0  TranslationROffsetUnits=m  TranslationZOffset=0  TranslationZOffsetUnits=m  TranslationThetaOffset=0  TranslationThetaOffsetUnits=deg  RotationMethod=StandardAxis  RotationAngleUnits=deg  RotationStandardAxis=+Y  RotationAngle=90  RotationArbitraryAxis=[0 0 1]  FollAlignAxisA=+X  BaseAlignAxisA=+Y  FollAlignAxisB=+Y  BaseAlignAxisB=+Z  RotationMatrix=[1 0 0; 0 1 0; 0 0 1]  BlockFunction=simmechanics.library.frames_transforms.rigid_transform
  Rigid Transform1 : sm_lib/Frames and Transforms/Rigid Transform  TranslationMethod=Cartesian  TranslationLengthUnit=m  TranslationStandardAxis=+Z  TranslationStandardOffset=0  TranslationCartesianOffset=pto.loc  TranslationROffset=0  TranslationROffsetUnits=m  TranslationZOffset=0  TranslationZOffsetUnits=m  TranslationThetaOffset=0  TranslationThetaOffsetUnits=deg  RotationMethod=StandardAxis  RotationAngleUnits=deg  RotationStandardAxis=+Y  RotationAngle=90  RotationArbitraryAxis=[0 0 1]  FollAlignAxisA=+X  BaseAlignAxisA=+Y  FollAlignAxisB=+Y  BaseAlignAxisB=+Z  RotationMatrix=[1 0 0; 0 1 0; 0 0 1]  BlockFunction=simmechanics.library.frames_transforms.rigid_transform
  Selector{,2,4,6} (4 alike) : Selector  InputPortWidth=3  Indices=[3 2 1]
  Selector{1,3,5,7} (4 alike) : Selector  InputPortWidth=3  Indices=[3]
  Simulink-PS Converter : nesl_utility/Simulink-PS Converter  PhysicalDomain=network_engine_domain  SubClassName=ps_input  LeftPortType=input  RightPortType=output  PseudoPeriodic=off  Frequencies=[]  NoiseDistribution=none  NoiseParameters=[]  Unit=1  AffineConversion=off  InputFiltering=derivs  SimscapeFilterOrder=2  InputFilterTimeConstant=0.001  UdotUserProvided=2
  Translational PCC (Prismatic Joint) : sm_lib/Joints/Prismatic Joint  SenseConstraintForce=on  SenseConstraintForceX=off  SenseConstraintForceY=off  SenseConstraintForceZ=off  SenseConstraintTorque=on  SenseConstraintTorqueX=off  SenseConstraintTorqueY=off  SenseConstraintTorqueZ=off  SenseTotalForce=on  SenseTotalForceX=off  SenseTotalForceY=off  SenseTotalForceZ=off  SenseTotalTorque=on  SenseTotalTorqueX=off  SenseTotalTorqueY=off  SenseTotalTorqueZ=off  CompositeWrenchDir=BaseOnFollower  CompositeWrenchFrame=BaseFrame  EquilibriumPosition=0  EquilibriumPositionUnits=m  SpringStiffness=pto.k  SpringStiffnessUnits=N/m  DampingCoefficient=pto.c  DampingCoefficientUnits=N/(m/s)  TorqueActuationMode=ComputedTorque  MotionActuationMode=InputMotion  SensePosition=on  SenseVelocity=on  SenseAcceleration=on  SenseTorqueForce=on  PositionTargetValue=0  PositionTargetValueUnits=m  PositionTargetSpecify=off  PositionTargetPriority=High  VelocityTargetValue=0  VelocityTargetValueUnits=m/s  VelocityTargetSpecify=off  VelocityTargetPriority=High  BlockFunction=simmechanics.library.joints.prismatic_joint
  output : ToWorkspace  VariableName=pto1_out  SaveFormat=Structure With Time  SampleTime=-1
  F : PMIOPort  Port=1  Side=Left
  B : PMIOPort  Port=2  Side=Right
  wires:
  Assignment (1st index)2/1 -> Mux2/3  "acceleration"
  Assignment (1st index)1/1 -> Mux2/2, ForceAndPower/2(Vel)  "velocity"
  "Assignment (1st index) "/1 -> Mux2/1, ForceAndPower/1(Pos)  "position"
  Selector2/1 -> Selector3/1, Assignment/1
  Selector3/1 -> Gai57/1
  Gai57/1 -> Assignment/2
  Selector/1 -> Selector1/1, Assignment1/1
  Selector1/1 -> Gain4/1
  Gain4/1 -> Assignment1/2
  ForceAndPower/2(Power) -> Mux2/8  "powerInternalMechanics"
  ForceAndPower/1(Force) -> Mux2/7  "forceInternalMechanics"
  Assignment (1st index)3/1 -> Mux2/5  "forceActuation"
  Mux3/1 -> Mux2/4  "forceTotal"
  Mux1/1 -> Mux2/6  "forceConstraint"
  Mux2/1 -> output/1
  PS-Simulink Converter4/1 -> Selector/1
  PS-Simulink Converter5/1 -> Selector2/1
  PS-Simulink Converter1/1 -> Gain1/1
  Constant/1 -> "Assignment (1st index) "/1
  PS-Simulink Converter/1 -> Gain/1
  Gain/1 -> "Assignment (1st index) "/2
  Constant1/1 -> Assignment (1st index)1/1
  Gain1/1 -> Assignment (1st index)1/2
  Constant2/1 -> Assignment (1st index)2/1
  Constant3/1 -> Assignment (1st index)3/1
  Gain2/1 -> Assignment (1st index)2/2
  PS-Simulink Converter2/1 -> Gain2/1
  PS-Simulink Converter3/1 -> Gain3/1
  Gain3/1 -> Assignment (1st index)3/2
  Assignment1/1 -> Mux1/1
  Assignment/1 -> Mux1/2
  Selector6/1 -> Assignment2/1, Selector7/1
  Selector7/1 -> Gai1/1
  Gai1/1 -> Assignment2/2
  Selector4/1 -> Assignment3/1, Selector5/1
  Selector5/1 -> Gain5/1
  Gain5/1 -> Assignment3/2
  PS-Simulink Converter6/1 -> Selector4/1
  PS-Simulink Converter7/1 -> Selector6/1
  Assignment3/1 -> Mux3/1
  Assignment2/1 -> Mux3/2
  position/1 -> Simulink-PS Converter/1
  velocity/1 -> Simulink-PS Converter/2
  acceleration/1 -> Simulink-PS Converter/3
  connections:
  Rigid Transform/LConn1 -- B/RConn1
  Rigid Transform/RConn1 -- Translational PCC (Prismatic Joint)/LConn1
  Rigid Transform1/LConn1 -- F/RConn1
  PS-Simulink Converter4/LConn1 -- Translational PCC (Prismatic Joint)/RConn6
  PS-Simulink Converter5/LConn1 -- Translational PCC (Prismatic Joint)/RConn7
  Translational PCC (Prismatic Joint)/RConn2 -- PS-Simulink Converter/LConn1
  Translational PCC (Prismatic Joint)/RConn3 -- PS-Simulink Converter1/LConn1
  Translational PCC (Prismatic Joint)/RConn4 -- PS-Simulink Converter2/LConn1
  Translational PCC (Prismatic Joint)/RConn1 -- Rigid Transform1/RConn1
  Translational PCC (Prismatic Joint)/RConn5 -- PS-Simulink Converter3/LConn1
  Translational PCC (Prismatic Joint)/RConn8 -- PS-Simulink Converter6/LConn1
  PS-Simulink Converter7/LConn1 -- Translational PCC (Prismatic Joint)/RConn9
  Simulink-PS Converter/RConn1 -- Translational PCC (Prismatic Joint)/LConn2

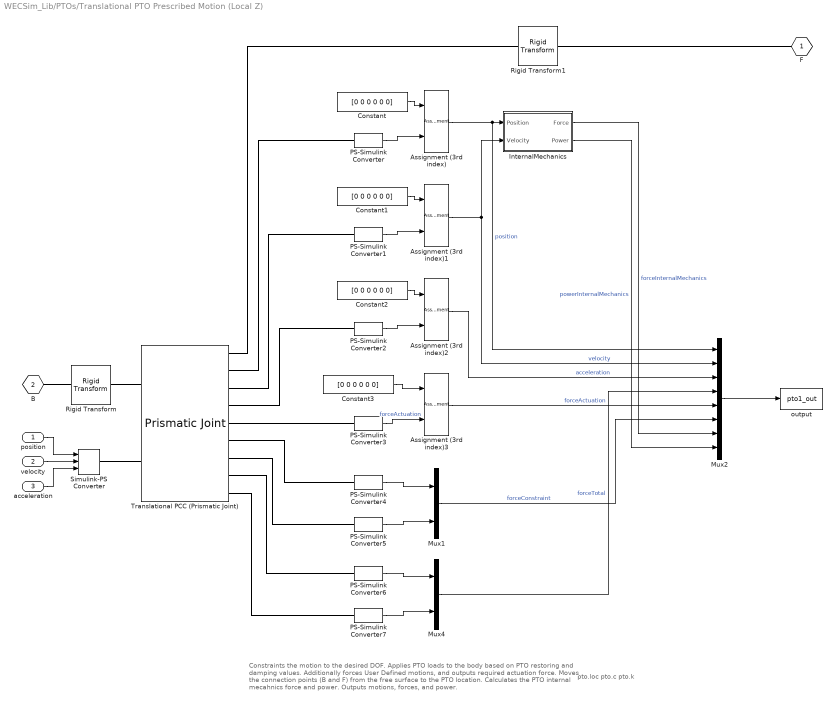
== system WECSim_Lib/PTOs/Translational PTO Prescribed Motion (Local Z) ==
  note: pto.loc
      | pto.c
      | pto.k
  note: Constraints the motion to the desired DOF.
      | Applies PTO loads to the body based on PTO restoring and damping values.
      | Additionally forces User Defined motions, and outputs required actuation force.
      | Moves the connection points (B and F) from the free surface to the PTO location.
      | Calculates the PTO internal mecahnics force and power.
      | Outputs motions, forces, and power.
  position : Inport
  velocity : Inport  Port=2
  acceleration : Inport  Port=3
  "Assignment (3rd index) " : Assignment  Indices=3
  Assignment (3rd index)1 : Assignment  Indices=3
  Assignment (3rd index)2 : Assignment  Indices=3
  Assignment (3rd index)3 : Assignment  Indices=3
  Constant{,1..3} (4 alike) : Constant  Value=[0 0 0 0 0 0]
  InternalMechanics : Subsystem
  Mux1 : Mux  Inputs=2
  Mux2 : Mux  Inputs=8
  Mux4 : Mux  Inputs=2
  PS-Simulink Converter{,1..7} (8 alike) : nesl_utility/PS-Simulink Converter  PhysicalDomain=network_engine_domain  SubClassName=ps_output  LeftPortType=input  RightPortType=output  PseudoPeriodic=off  Frequencies=[]  Unit=1  AffineConversion=off
  Rigid Transform : sm_lib/Frames and Transforms/Rigid Transform  TranslationMethod=Cartesian  TranslationLengthUnit=m  TranslationStandardAxis=+Z  TranslationStandardOffset=0  TranslationCartesianOffset=pto.loc  TranslationROffset=0  TranslationROffsetUnits=m  TranslationZOffset=0  TranslationZOffsetUnits=m  TranslationThetaOffset=0  TranslationThetaOffsetUnits=deg  RotationMethod=None  RotationAngleUnits=deg  RotationStandardAxis=+X  RotationAngle=90  RotationArbitraryAxis=[0 0 1]  FollAlignAxisA=+X  BaseAlignAxisA=+Y  FollAlignAxisB=+Y  BaseAlignAxisB=+Z  RotationMatrix=[1 0 0; 0 1 0; 0 0 1]  BlockFunction=simmechanics.library.frames_transforms.rigid_transform
  Rigid Transform1 : sm_lib/Frames and Transforms/Rigid Transform  TranslationMethod=Cartesian  TranslationLengthUnit=m  TranslationStandardAxis=+Z  TranslationStandardOffset=0  TranslationCartesianOffset=pto.loc  TranslationROffset=0  TranslationROffsetUnits=m  TranslationZOffset=0  TranslationZOffsetUnits=m  TranslationThetaOffset=0  TranslationThetaOffsetUnits=deg  RotationMethod=None  RotationAngleUnits=deg  RotationStandardAxis=+X  RotationAngle=90  RotationArbitraryAxis=[0 0 1]  FollAlignAxisA=+X  BaseAlignAxisA=+Y  FollAlignAxisB=+Y  BaseAlignAxisB=+Z  RotationMatrix=[1 0 0; 0 1 0; 0 0 1]  BlockFunction=simmechanics.library.frames_transforms.rigid_transform
  Simulink-PS Converter : nesl_utility/Simulink-PS Converter  PhysicalDomain=network_engine_domain  SubClassName=ps_input  LeftPortType=input  RightPortType=output  PseudoPeriodic=off  Frequencies=[]  NoiseDistribution=none  NoiseParameters=[]  Unit=1  AffineConversion=off  InputFiltering=derivs  SimscapeFilterOrder=2  InputFilterTimeConstant=0.001  UdotUserProvided=2
  Translational PCC (Prismatic Joint) : sm_lib/Joints/Prismatic Joint  SenseConstraintForce=on  SenseConstraintForceX=off  SenseConstraintForceY=off  SenseConstraintForceZ=off  SenseConstraintTorque=on  SenseConstraintTorqueX=off  SenseConstraintTorqueY=off  SenseConstraintTorqueZ=off  SenseTotalForce=on  SenseTotalForceX=off  SenseTotalForceY=off  SenseTotalForceZ=off  SenseTotalTorque=on  SenseTotalTorqueX=off  SenseTotalTorqueY=off  SenseTotalTorqueZ=off  CompositeWrenchDir=BaseOnFollower  CompositeWrenchFrame=BaseFrame  EquilibriumPosition=0  EquilibriumPositionUnits=m  SpringStiffness=pto.k  SpringStiffnessUnits=N/m  DampingCoefficient=pto.c  DampingCoefficientUnits=N/(m/s)  TorqueActuationMode=ComputedTorque  MotionActuationMode=InputMotion  SensePosition=on  SenseVelocity=on  SenseAcceleration=on  SenseTorqueForce=on  PositionTargetValue=0  PositionTargetValueUnits=m  PositionTargetSpecify=off  PositionTargetPriority=High  VelocityTargetValue=0  VelocityTargetValueUnits=m/s  VelocityTargetSpecify=off  VelocityTargetPriority=High  BlockFunction=simmechanics.library.joints.prismatic_joint
  output : ToWorkspace  VariableName=pto1_out  SaveFormat=Structure With Time  SampleTime=-1
  F : PMIOPort  Port=1  Side=Left
  B : PMIOPort  Port=2  Side=Right
  wires:
  PS-Simulink Converter3/1 -> Assignment (3rd index)3/2  "forceActuation"
  Constant3/1 -> Assignment (3rd index)3/1
  InternalMechanics/2(Power) -> Mux2/8  "powerInternalMechanics"
  InternalMechanics/1(Force) -> Mux2/7  "forceInternalMechanics"
  PS-Simulink Converter2/1 -> Assignment (3rd index)2/2
  Constant2/1 -> Assignment (3rd index)2/1
  PS-Simulink Converter1/1 -> Assignment (3rd index)1/2
  Constant1/1 -> Assignment (3rd index)1/1
  PS-Simulink Converter/1 -> "Assignment (3rd index) "/2
  Constant/1 -> "Assignment (3rd index) "/1
  Assignment (3rd index)2/1 -> Mux2/3  "acceleration"
  Assignment (3rd index)1/1 -> InternalMechanics/2(Velocity), Mux2/2  "velocity"
  "Assignment (3rd index) "/1 -> InternalMechanics/1(Position), Mux2/1  "position"
  Assignment (3rd index)3/1 -> Mux2/5  "forceActuation"
  PS-Simulink Converter7/1 -> Mux4/2
  PS-Simulink Converter6/1 -> Mux4/1
  PS-Simulink Converter5/1 -> Mux1/2
  PS-Simulink Converter4/1 -> Mux1/1
  Mux4/1 -> Mux2/4  "forceTotal"
  Mux1/1 -> Mux2/6  "forceConstraint"
  Mux2/1 -> output/1
  position/1 -> Simulink-PS Converter/1
  velocity/1 -> Simulink-PS Converter/2
  acceleration/1 -> Simulink-PS Converter/3
  connections:
  Translational PCC (Prismatic Joint)/RConn9 -- PS-Simulink Converter7/LConn1
  Translational PCC (Prismatic Joint)/RConn8 -- PS-Simulink Converter6/LConn1
  Translational PCC (Prismatic Joint)/RConn7 -- PS-Simulink Converter5/LConn1
  Translational PCC (Prismatic Joint)/RConn6 -- PS-Simulink Converter4/LConn1
  Translational PCC (Prismatic Joint)/RConn5 -- PS-Simulink Converter3/LConn1
  Translational PCC (Prismatic Joint)/RConn4 -- PS-Simulink Converter2/LConn1
  Translational PCC (Prismatic Joint)/RConn3 -- PS-Simulink Converter1/LConn1
  Translational PCC (Prismatic Joint)/RConn2 -- PS-Simulink Converter/LConn1
  B/RConn1 -- Rigid Transform/LConn1
  Rigid Transform/RConn1 -- Translational PCC (Prismatic Joint)/LConn1
  Translational PCC (Prismatic Joint)/RConn1 -- Rigid Transform1/RConn1
  Rigid Transform1/LConn1 -- F/RConn1
  Translational PCC (Prismatic Joint)/LConn2 -- Simulink-PS Converter/RConn1
